simulink model "filtrage_Simulink__DSP_toolbox"  (R2019b)
settings: Solver=VariableStepAuto  StartTime=0.0  StopTime=10.0  RelTol=1e-3
InitFcn:
  | load filtrage_pb_ordre_1.mat;
libraries: dsparch4 x1
settings Model: Creator=ivanl  LastModifiedBy=ivanl

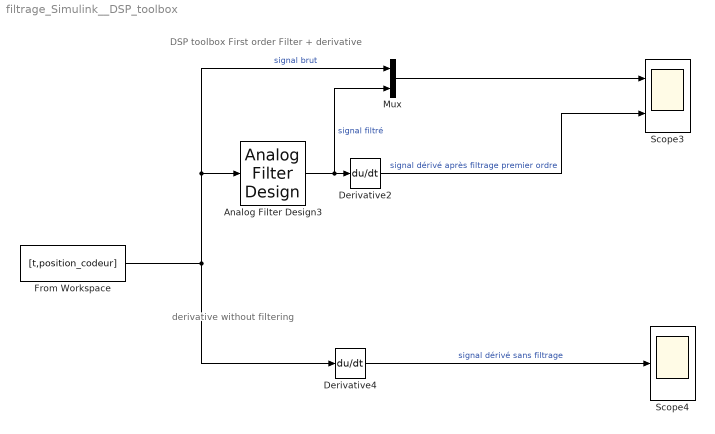
== system filtrage_Simulink__DSP_toolbox ==
  note: derivative without filtering
  note: DSP toolbox First order Filter + derivative
  Analog Filter Design3 : dsparch4/Analog Filter Design  method=Butterworth  filttype=Lowpass  N=1  Wlo=5  Whi=80  Rp=2  Rs=40
  Derivative2 : Derivative
  Derivative4 : Derivative
  From Workspace : FromWorkspace  VariableName=[t,position_codeur]  SampleTime=0.001
  Mux : Mux  Inputs=2
  Scope3 : Scope  NumInputPorts=2
  Scope4 : Scope
  wires:
  Analog Filter Design3/1 -> Derivative2/1, Mux/2  "signal filtré"
  Derivative2/1 -> Scope3/2  "signal dérivé après filtrage premier ordre"
  Mux/1 -> Scope3/1
  Derivative4/1 -> Scope4/1  "signal dérivé sans filtrage"
  From Workspace/1 -> Derivative4/1, Mux/1, Analog Filter Design3/1  "signal brut"
